simulink model "control_sipro_b35"  (R2018a)
settings: Solver=VariableStepAuto  StartTime=0.0  StopTime=10.0  RelTol=1e-3
values from neighbouring files (symbols this model uses):
  A = [0 1; -4 0]    [main.m]
  B = [0 ; 4]    [main.m]
  C = [1, 0]    [main.m]
  D = 0    [main.m]
  den = [1 0 4]    [main.m]
  num = [w0*w0*G]    [main.m]
undefined symbols (not defined in the file or in its folder): atilde, btilde
settings Model: Creator=Sampreet Sarkar  LastModifiedBy=Sampreet Sarkar

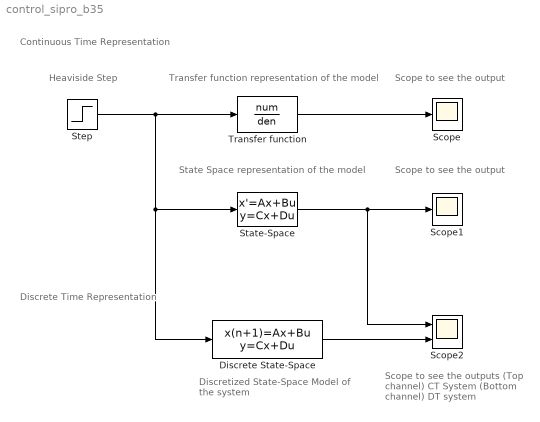
== system control_sipro_b35 ==
  note: Discrete Time Representation
  note: Scope to see the outputs
      | (Top channel) CT System
      | (Bottom channel) DT system
  note: Discretized State-Space Model
      | of the system
  note: Continuous Time Representation
  note: Scope to see the output
  note: Heaviside Step
  note: Transfer function representation of the model
  note: Scope to see the output
  note: State Space representation of the model
  Discrete State-Space : DiscreteStateSpace  A=atilde  B=btilde  C=C  D=D  SampleTime=-1
  Scope : Scope
  Scope1 : Scope
  Scope2 : Scope  NumInputPorts=2
  State-Space : StateSpace  A=A  B=B  C=C  D=D  InitialCondition=0
  Step : Step  After=0.05  SampleTime=0
  "Transfer function " : TransferFcn  Numerator=num  Denominator=den
  wires:
  "Transfer function "/1 -> Scope/1
  Step/1 -> Discrete State-Space/1, State-Space/1, "Transfer function "/1
  State-Space/1 -> Scope2/1, Scope1/1
  Discrete State-Space/1 -> Scope2/2
